simulink model "DIesi1"  (R2020a)
settings: Solver=ode4  StartTime=0.0  StopTime=5e-4  FixedStep=1e-8  RelTol=1e-6  AbsTol=1e-6
InitFcn:
  | R1 = 1000;
  | R2 = 20;
  | L = 25.3E-6;
  | C = 100E-9;
  | IS = 1E-8;
  | UT = 26E-3;
  | f = 0.15E+6;
settings Model: Creator=LKP  LastModifiedBy=peter
settings DataIOCC: OutputOption=SpecifiedOutputTimes  OutputTimes=0:1e-8:5e-4

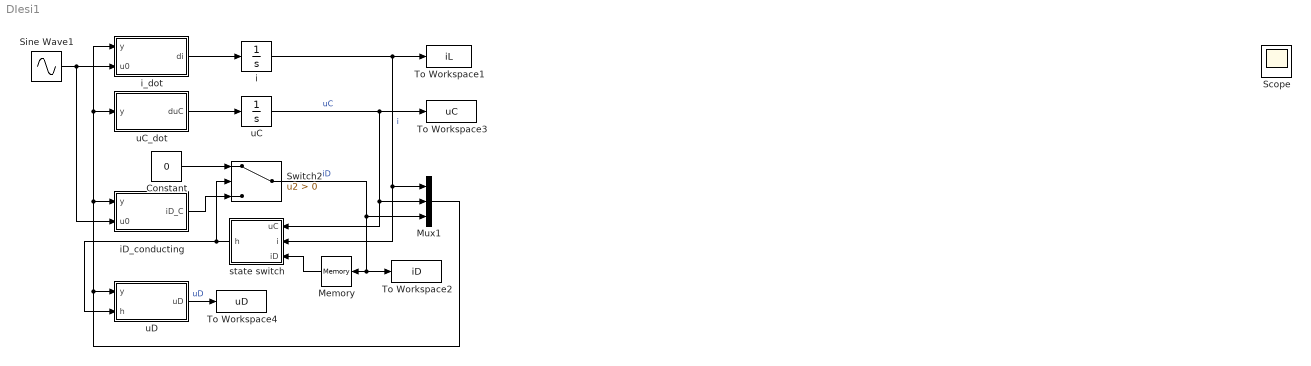
== system DIesi1 ==
  Constant : Constant  Value=0
  Memory : Memory
  Mux1 : Mux  Inputs=3
  Sine Wave1 : Sin  Amplitude=-1  Frequency=2*pi*f  SampleTime=0
  Switch2 : Switch  Criteria=u2 > Threshold
  To Workspace1 : ToWorkspace  VariableName=iL  SaveFormat=Timeseries  SampleTime=-1
  To Workspace2 : ToWorkspace  VariableName=iD  SaveFormat=Timeseries  SampleTime=-1
  To Workspace3 : ToWorkspace  VariableName=uC  SaveFormat=Timeseries  SampleTime=-1
  To Workspace4 : ToWorkspace  VariableName=uD  SaveFormat=Timeseries  SampleTime=-1
  i : Integrator
  iD_conducting : Subsystem
  i_dot : Subsystem
  state switch : Subsystem
  uC : Integrator
  uC_dot : Subsystem
  uD : Subsystem
  Scope : Scope
  wires:
  uC/1 -> To Workspace3/1, Mux1/2, state switch/1(uC)  "uC"
  i/1 -> To Workspace1/1, Mux1/1, state switch/2(i)  "i"
  Mux1/1 -> uD/1(y), i_dot/1(y), uC_dot/1(y), iD_conducting/1(y)
  i_dot/1(di) -> i/1
  uC_dot/1(duC) -> uC/1
  state switch/1(h) -> uD/2(h), Switch2/2
  Constant/1 -> Switch2/1
  iD_conducting/1(iD_C) -> Switch2/3
  Switch2/1 -> Mux1/3, To Workspace2/1, Memory/1  "iD"
  Memory/1 -> state switch/3(iD)
  Sine Wave1/1 -> iD_conducting/2(u0), i_dot/2(u0)
  uD/1(uD) -> To Workspace4/1  "uD"

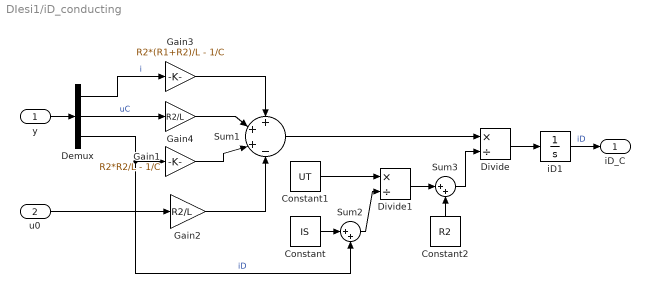
== system DIesi1/iD_conducting ==
  y : Inport
  u0 : Inport  Port=2
  Constant : Constant  Value=IS
  Constant1 : Constant  Value=UT
  Constant2 : Constant  Value=R2
  Demux : Demux  Outputs=3
  Divide : Product  Inputs=*/
  Divide1 : Product  Inputs=*/
  Gain1 : Gain  Gain=R2*R2/L - 1/C
  Gain2 : Gain  Gain=R2/L
  Gain3 : Gain  Gain=R2*(R1+R2)/L - 1/C
  Gain4 : Gain  Gain=R2/L
  Sum1 : Sum  Inputs=+++-
  Sum2 : Sum  Inputs=|++
  Sum3 : Sum  Inputs=|++
  iD1 : Integrator
  iD_C : Outport
  wires:
  y/1 -> Demux/1
  u0/1 -> Gain2/1
  iD1/1 -> iD_C/1  "iD"
  Demux/1 -> Gain3/1  "i"
  Demux/3 -> Sum2/2, Gain1/1  "iD"
  Demux/2 -> Gain4/1  "uC"
  Gain3/1 -> Sum1/1
  Gain4/1 -> Sum1/2
  Gain1/1 -> Sum1/3
  Sum1/1 -> Divide/1
  Constant/1 -> Sum2/1
  Constant1/1 -> Divide1/1
  Sum2/1 -> Divide1/2
  Divide1/1 -> Sum3/1
  Constant2/1 -> Sum3/2
  Sum3/1 -> Divide/2
  Divide/1 -> iD1/1
  Gain2/1 -> Sum1/4

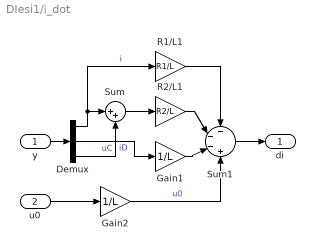
== system DIesi1/i_dot ==
  y : Inport
  u0 : Inport  Port=2
  Demux : Demux  Outputs=3
  Gain1 : Gain  Gain=1/L
  Gain2 : Gain  Gain=1/L
  R1/L1 : Gain  Gain=R1/L
  R2/L1 : Gain  Gain=R2/L
  Sum : Sum  Inputs=|++
  Sum1 : Sum  Inputs=---+
  di : Outport
  wires:
  y/1 -> Demux/1
  Demux/1 -> R1/L1/1, Sum/1  "i"
  Sum/1 -> R2/L1/1
  Demux/2 -> Gain1/1  "uC"
  R1/L1/1 -> Sum1/1
  R2/L1/1 -> Sum1/2
  Gain1/1 -> Sum1/3
  Gain2/1 -> Sum1/4  "u0"
  Sum1/1 -> di/1
  Demux/3 -> Sum/2  "iD"
  u0/1 -> Gain2/1

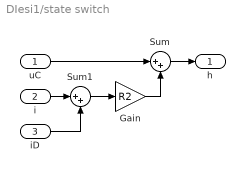
== system DIesi1/state switch ==
  uC : Inport
  i : Inport  Port=2
  iD : Inport  Port=3
  Gain : Gain  Gain=R2
  Sum : Sum  Inputs=|++
  Sum1 : Sum  Inputs=|++
  h : Outport
  wires:
  uC/1 -> Sum/1
  Sum/1 -> h/1
  Gain/1 -> Sum/2
  i/1 -> Sum1/1
  Sum1/1 -> Gain/1
  iD/1 -> Sum1/2

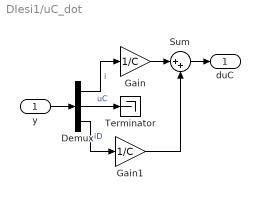
== system DIesi1/uC_dot ==
  y : Inport
  Demux : Demux  Outputs=3
  Gain : Gain  Gain=1/C
  Gain1 : Gain  Gain=1/C
  Sum : Sum  Inputs=|++
  Terminator : Terminator
  duC : Outport
  wires:
  Gain/1 -> Sum/1
  Sum/1 -> duC/1
  y/1 -> Demux/1
  Demux/1 -> Gain/1  "i"
  Demux/2 -> Terminator/1  "uC"
  Demux/3 -> Gain1/1  "iD"
  Gain1/1 -> Sum/2

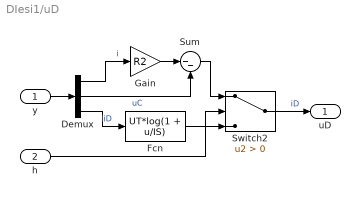
== system DIesi1/uD ==
  y : Inport
  h : Inport  Port=2
  Demux : Demux  Outputs=3
  Fcn : Fcn  Expr=UT*log(1 + u/IS)
  Gain : Gain  Gain=R2
  Sum : Sum  Inputs=|--
  Switch2 : Switch  Criteria=u2 > Threshold
  uD : Outport
  wires:
  Switch2/1 -> uD/1  "iD"
  h/1 -> Switch2/2
  Sum/1 -> Switch2/1
  y/1 -> Demux/1
  Demux/1 -> Gain/1  "i"
  Demux/2 -> Sum/2  "uC"
  Demux/3 -> Fcn/1  "iD"
  Gain/1 -> Sum/1
  Fcn/1 -> Switch2/3
